simulink subsystem "Adapter"  (R2023a)
settings: Solver=VariableStepAuto  StartTime=0.0  StopTime=10.0  RelTol=1e-3
libraries: simulink x1
settings Model: Creator=lehas  LastModifiedBy=lehas

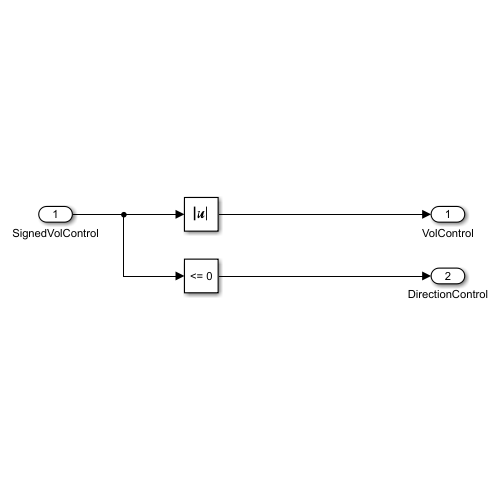
[thumbnail: Simulink's stored preview of the top-level diagram]
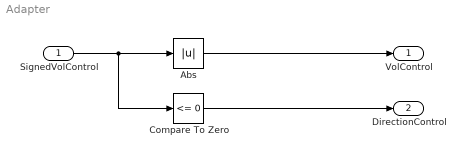
== system Adapter ==
  SignedVolControl : Inport
  Abs : Abs  SaturateOnIntegerOverflow=off
  Compare To Zero : simulink/Logic and Bit Operations/Compare To Zero  relop=<=  OutDataTypeStr=boolean
  VolControl : Outport
  DirectionControl : Outport  Port=2  OutDataTypeStr=boolean
  wires:
  SignedVolControl/1 -> Compare To Zero/1, Abs/1
  Abs/1 -> VolControl/1
  Compare To Zero/1 -> DirectionControl/1
